simulink model "mrefrobotarm_modified_previous_y_previous_u_previous_ref_pert_2"  (R2018b)
settings: Solver=FixedStepAuto  StartTime=0.0  StopTime=60  RelTol=1e-3  AbsTol=1e-6
undefined symbols (not defined in the file or in its folder): cc, options
libraries: neural x858, simulink x1
(part 24 of 32)

== system mrefrobotarm_modified_previous_y_previous_u_previous_ref_pert_2/m=0.001 sd=0.001/Layer 3/Delays 1 ==
  "p{3}" : Inport  PortDimensions=30
      mask Display: e = 0.06;c1 = [120 230 180]/255;c2 = ([120 230 180]+0)/(256+128);c3 = ([120 230 180]+128)/(256+128);patch([0 1 1 0],[0 0 1 1],c1);patch([0 1 1 1-e 1-e 0+e],[0 0 1 1-e 0+e 0+e],c2);patch([0 0 1 1-e 0+e 0+e],[0 1 1 1-e 1-e 0+e],c3);plot([0 1 1 0 0],[0 0 1 1 0]);
  mux : Mux  Inputs=1
      mask Display: e = 0.06;c1 = [120 150 230]/255;c2 = ([120 150 230]+0)/383;c3 = ([120 150 230]+128)/383;patch([0 1 1 0],[0 0 1 1],c1);patch([0 1 1 1-e 1-e 0+e],[0 0 1 1-e 0+e 0+e],c2);patch([0 0 1 1-e 0+e 0+e],[0 1 1 1-e 1-e 0+e],c3);plot([0 1 1 0 0],[0 0 1 1 0]);disp('Mux')
  "pd{3,2}" : Outport
      mask Display: e = 0.06;c1 = [120 230 180]/255;c2 = ([120 230 180]+0)/(256+128);c3 = ([120 230 180]+128)/(256+128);patch([0 1 1 0],[0 0 1 1],c1);patch([0 1 1 1-e 1-e 0+e],[0 0 1 1-e 0+e 0+e],c2);patch([0 0 1 1-e 0+e 0+e],[0 1 1 1-e 1-e 0+e],c3);plot([0 1 1 0 0],[0 0 1 1 0]);
  wires:
  "p{3}"/1 -> mux/1
  mux/1 -> "pd{3,2}"/1

== system mrefrobotarm_modified_previous_y_previous_u_previous_ref_pert_2/m=0.001 sd=0.001/Layer 3/LW{3,2} ==
  "ad{3,2}" : Inport  PortDimensions=30
      mask Display: e = 0.06;c1 = [120 230 180]/255;c2 = ([120 230 180]+0)/(256+128);c3 = ([120 230 180]+128)/(256+128);patch([0 1 1 0],[0 0 1 1],c1);patch([0 1 1 1-e 1-e 0+e],[0 0 1 1-e 0+e 0+e],c2);patch([0 0 1 1-e 0+e 0+e],[0 1 1 1-e 1-e 0+e],c3);plot([0 1 1 0 0],[0 0 1 1 0]);
  "IW{3,2}(1,:)'" : Constant  Value=[-0.00096598592137593663510541919237084584892727434635162353515625;-0.03126267992859599331723075010813772678375244140625;-0.00195354501463004294470326982491314993239939212799072265625;-0.047903518138686769500811379884908092208206653594970703125;-0.0230636981987975865637796601959053077735006809234619140625;0.1680979203439105507111861470548319630324840545654296875;-0.0023952928575741243809316127766351200989447534084320068359375;0.0088298450217599577793947673853836022317409515380859375;0.00448404494478483149622061176842180429957807064056396484375;0.07350633081296938098336823941281181760132312774658203125;0.004624123527908109536344039014466034132055938243865966796875;0.03743489095666606425449884909539832733571529388427734375;-0.12573771491850338488660554503439925611019134521484375;-0.07859633251545668219950613320179400034248828887939453125;0.005914082534642393917945213388520642183721065521240234375;0.0135763042468372945037469179396794061176478862762451171875;0.0154239171401948822748284584349676151759922504425048828125;-0.007373815499766849142215807688671702635474503040313720703125;0.001608015075631823685708976512387380353175103664398193359375;0.0603517965756205920779819962262990884482860565185546875;-0.77977075469641288218980434976401738822460174560546875;0.85569988582330436255318772964528761804103851318359375;0.01259027748586210616876801537955543608404695987701416015625;-0.003409584380003004115688991504384830477647483348846435546875;-0.03508176609962354586258470590109936892986297607421875;0.0153176587784085542487400033451194758526980876922607421875;0.053023670382310893189892198051893501542508602142333984375;-0.0218811595943164440003503301568343886174261569976806640625;-0.0679133358367276229738962456394801847636699676513671875;0.1352169568786299180818133436332573182880878448486328125]
      mask Display: e = 0.06;c1 = [120 150 230]/255;c2 = ([120 150 230]+0)/383;c3 = ([120 150 230]+128)/383;patch([0 1 1 0],[0 0 1 1],c1);patch([0 1 1 1-e 1-e 0+e],[0 0 1 1-e 0+e 0+e],c2);patch([0 0 1 1-e 0+e 0+e],[0 1 1 1-e 1-e 0+e],c3);plot([0 1 1 0 0],[0 0 1 1 0]);disp('weights');
  Mux : Mux  Inputs=1
      mask Display: e = 0.06;c1 = [120 150 230]/255;c2 = ([120 150 230]+0)/383;c3 = ([120 150 230]+128)/383;patch([0 1 1 0],[0 0 1 1],c1);patch([0 1 1 1-e 1-e 0+e],[0 0 1 1-e 0+e 0+e],c2);patch([0 0 1 1-e 0+e 0+e],[0 1 1 1-e 1-e 0+e],c3);plot([0 1 1 0 0],[0 0 1 1 0]);disp('Mux');
  dotprod1 : neural/Weight Functions/dotprod
  "lz{3,2}" : Outport
      mask Display: e = 0.06;c1 = [120 230 180]/255;c2 = ([120 230 180]+0)/(256+128);c3 = ([120 230 180]+128)/(256+128);patch([0 1 1 0],[0 0 1 1],c1);patch([0 1 1 1-e 1-e 0+e],[0 0 1 1-e 0+e 0+e],c2);patch([0 0 1 1-e 0+e 0+e],[0 1 1 1-e 1-e 0+e],c3);plot([0 1 1 0 0],[0 0 1 1 0]);
  wires:
  "IW{3,2}(1,:)'"/1 -> dotprod1/1
  "ad{3,2}"/1 -> dotprod1/2
  dotprod1/1 -> Mux/1
  Mux/1 -> "lz{3,2}"/1

== system mrefrobotarm_modified_previous_y_previous_u_previous_ref_pert_2/m=0.001 sd=0.001 unclear/Layer 1/Delays 1 ==
  "p{1}" : Inport  PortDimensions=10
      mask Display: e = 0.06;c1 = [120 230 180]/255;c2 = ([120 230 180]+0)/(256+128);c3 = ([120 230 180]+128)/(256+128);patch([0 1 1 0],[0 0 1 1],c1);patch([0 1 1 1-e 1-e 0+e],[0 0 1 1-e 0+e 0+e],c2);patch([0 0 1 1-e 0+e 0+e],[0 1 1 1-e 1-e 0+e],c3);plot([0 1 1 0 0],[0 0 1 1 0]);
  mux : Mux  Inputs=1
      mask Display: e = 0.06;c1 = [120 150 230]/255;c2 = ([120 150 230]+0)/383;c3 = ([120 150 230]+128)/383;patch([0 1 1 0],[0 0 1 1],c1);patch([0 1 1 1-e 1-e 0+e],[0 0 1 1-e 0+e 0+e],c2);patch([0 0 1 1-e 0+e 0+e],[0 1 1 1-e 1-e 0+e],c3);plot([0 1 1 0 0],[0 0 1 1 0]);disp('Mux')
  "pd{1,1}" : Outport
      mask Display: e = 0.06;c1 = [120 230 180]/255;c2 = ([120 230 180]+0)/(256+128);c3 = ([120 230 180]+128)/(256+128);patch([0 1 1 0],[0 0 1 1],c1);patch([0 1 1 1-e 1-e 0+e],[0 0 1 1-e 0+e 0+e],c2);patch([0 0 1 1-e 0+e 0+e],[0 1 1 1-e 1-e 0+e],c3);plot([0 1 1 0 0],[0 0 1 1 0]);
  wires:
  "p{1}"/1 -> mux/1
  mux/1 -> "pd{1,1}"/1

== system mrefrobotarm_modified_previous_y_previous_u_previous_ref_pert_2/m=0.001 sd=0.001 unclear/Layer 1/IW{1,1} ==
  "pd{1,1}" : Inport  PortDimensions=10
      mask Display: e = 0.06;c1 = [120 230 180]/255;c2 = ([120 230 180]+0)/(256+128);c3 = ([120 230 180]+128)/(256+128);patch([0 1 1 0],[0 0 1 1],c1);patch([0 1 1 1-e 1-e 0+e],[0 0 1 1-e 0+e 0+e],c2);patch([0 0 1 1-e 0+e 0+e],[0 1 1 1-e 1-e 0+e],c3);plot([0 1 1 0 0],[0 0 1 1 0]);
  "IW{1,1}(1,:)'" : Constant  Value=[0.350735520146514712092056242909166030585765838623046875;-0.365382843268743207065796241295174695551395416259765625;-0.99622776359163045523104074163711629807949066162109375;-0.2204237782535651835047474378370679914951324462890625;-1.1029132366021070499328970981878228485584259033203125;0.1267678513277864238428804810610017739236354827880859375;0.11285976385185104986508264346412033773958683013916015625;0.0266590202247262118839810085546560003422200679779052734375;1.4467040095656533704726598443812690675258636474609375;1.3454075388999766627051712930551730096340179443359375]
      mask Display: e = 0.06;c1 = [120 150 230]/255;c2 = ([120 150 230]+0)/383;c3 = ([120 150 230]+128)/383;patch([0 1 1 0],[0 0 1 1],c1);patch([0 1 1 1-e 1-e 0+e],[0 0 1 1-e 0+e 0+e],c2);patch([0 0 1 1-e 0+e 0+e],[0 1 1 1-e 1-e 0+e],c3);plot([0 1 1 0 0],[0 0 1 1 0]);disp('Weights');
  "IW{1,1}(10,:)'" : Constant  Value=[0.489180396685796214928387826148536987602710723876953125;0.025688296059734945508967740579464589245617389678955078125;-0.8253001755471967015864720451645553112030029296875;-0.3423875044746698126374440107611007988452911376953125;2.30371194741592777432970251538790762424468994140625;-3.4241648689344543754486949183046817779541015625;1.3873334301899580278671919586486183106899261474609375;-0.44829248082369443917372109353891573846340179443359375;-0.584485848536391738861084377276711165904998779296875;-0.78044816092502511395423425710760056972503662109375]
      mask Display: e = 0.06;c1 = [120 150 230]/255;c2 = ([120 150 230]+0)/383;c3 = ([120 150 230]+128)/383;patch([0 1 1 0],[0 0 1 1],c1);patch([0 1 1 1-e 1-e 0+e],[0 0 1 1-e 0+e 0+e],c2);patch([0 0 1 1-e 0+e 0+e],[0 1 1 1-e 1-e 0+e],c3);plot([0 1 1 0 0],[0 0 1 1 0]);disp('Weights');
  "IW{1,1}(11,:)'" : Constant  Value=[0.18698885547596300060746443705284036695957183837890625;0.93870062216768701546243391931056976318359375;-0.87771687606838610928861044158111326396465301513671875;0.525629157232238686248138037626631557941436767578125;-0.584803275112354636888767345226369798183441162109375;-0.78398570882191587205767291379743255674839019775390625;-0.6750269388772991430158754155854694545269012451171875;-0.037333925850436155968736784416250884532928466796875;-1.1760354680013247463676862025749869644641876220703125;-0.3408361228029785916504579290631227195262908935546875]
      mask Display: e = 0.06;c1 = [120 150 230]/255;c2 = ([120 150 230]+0)/383;c3 = ([120 150 230]+128)/383;patch([0 1 1 0],[0 0 1 1],c1);patch([0 1 1 1-e 1-e 0+e],[0 0 1 1-e 0+e 0+e],c2);patch([0 0 1 1-e 0+e 0+e],[0 1 1 1-e 1-e 0+e],c3);plot([0 1 1 0 0],[0 0 1 1 0]);disp('Weights');
  "IW{1,1}(12,:)'" : Constant  Value=[0.0215852682713452322105229796989078749902546405792236328125;-0.51872830046918327884242216896382160484790802001953125;-0.468248523931060589564623342084814794361591339111328125;-0.50647243936863173274787186528556048870086669921875;-0.78157350595780050728222931866184808313846588134765625;3.41692574461050213585622259415686130523681640625;-2.23846059049971923826660713530145585536956787109375;-0.60927422485717841471597466806997545063495635986328125;0.29327799124264597452338421135209500789642333984375;0.08903506975016380053933318095005233772099018096923828125]
      mask Display: e = 0.06;c1 = [120 150 230]/255;c2 = ([120 150 230]+0)/383;c3 = ([120 150 230]+128)/383;patch([0 1 1 0],[0 0 1 1],c1);patch([0 1 1 1-e 1-e 0+e],[0 0 1 1-e 0+e 0+e],c2);patch([0 0 1 1-e 0+e 0+e],[0 1 1 1-e 1-e 0+e],c3);plot([0 1 1 0 0],[0 0 1 1 0]);disp('Weights');
  "IW{1,1}(13,:)'" : Constant  Value=[0.6746875013157798139928900127415545284748077392578125;-0.62489238655318668502758328031632117927074432373046875;0.1629262490629680704135040514302090741693973541259765625;-0.1367019703160116950169111760260420851409435272216796875;-0.75570950017347160443392795059480704367160797119140625;2.003318792327748010251298182993195950984954833984375;-1.1536359129580089355471272938302718102931976318359375;-0.041927729311054200145303383351347292773425579071044921875;0.843791037259761456112983069033361971378326416015625;1.0843679220652264749702453627833165228366851806640625]
      mask Display: e = 0.06;c1 = [120 150 230]/255;c2 = ([120 150 230]+0)/383;c3 = ([120 150 230]+128)/383;patch([0 1 1 0],[0 0 1 1],c1);patch([0 1 1 1-e 1-e 0+e],[0 0 1 1-e 0+e 0+e],c2);patch([0 0 1 1-e 0+e 0+e],[0 1 1 1-e 1-e 0+e],c3);plot([0 1 1 0 0],[0 0 1 1 0]);disp('Weights');
  "IW{1,1}(14,:)'" : Constant  Value=[0.1064105997657826818691972903252462856471538543701171875;-0.76827006137680131647726966548361815512180328369140625;1.186307378378237853411292235250584781169891357421875;0.56761102937644825061624942463822662830352783203125;-1.5212597719010518826365796485333703458309173583984375;1.5024445400946202511249794042669236660003662109375;-1.3109166464008394914486643756390549242496490478515625;0.08636767886193663645855167487752623856067657470703125;-1.7985044176385340808366208875668235123157501220703125;-0.31523953859487263695626779735903255641460418701171875]
      mask Display: e = 0.06;c1 = [120 150 230]/255;c2 = ([120 150 230]+0)/383;c3 = ([120 150 230]+128)/383;patch([0 1 1 0],[0 0 1 1],c1);patch([0 1 1 1-e 1-e 0+e],[0 0 1 1-e 0+e 0+e],c2);patch([0 0 1 1-e 0+e 0+e],[0 1 1 1-e 1-e 0+e],c3);plot([0 1 1 0 0],[0 0 1 1 0]);disp('Weights');
  "IW{1,1}(15,:)'" : Constant  Value=[-0.281470768776616087070152616433915682137012481689453125;1.3938473337264507545540936916950158774852752685546875;-1.0094685935062079895629949533031322062015533447265625;-0.462216053281385708118023103452287614345550537109375;-2.023964996515461134407587451278232038021087646484375;0.488549499659554575803355191965238191187381744384765625;0.67736367905604721872947493466199375689029693603515625;0.340098821019820307665071368319331668317317962646484375;0.82710042766707292383188132589566521346569061279296875;0.03264495933566601004738316760267480276525020599365234375]
      mask Display: e = 0.06;c1 = [120 150 230]/255;c2 = ([120 150 230]+0)/383;c3 = ([120 150 230]+128)/383;patch([0 1 1 0],[0 0 1 1],c1);patch([0 1 1 1-e 1-e 0+e],[0 0 1 1-e 0+e 0+e],c2);patch([0 0 1 1-e 0+e 0+e],[0 1 1 1-e 1-e 0+e],c3);plot([0 1 1 0 0],[0 0 1 1 0]);disp('Weights');
  "IW{1,1}(16,:)'" : Constant  Value=[0.51236814799393159969298494615941308438777923583984375;-0.11271288636420510875790768068327452056109905242919921875;-0.86745597821140341121548544833785854279994964599609375;-0.0444761804672831051465919927068171091377735137939453125;0.292548210338565983779091084215906448662281036376953125;1.1887786529416064507103101277607493102550506591796875;-1.5965228644647548872370634853723458945751190185546875;-0.1933031790978570196859465113448095507919788360595703125;1.653612394779674144018599690753035247325897216796875;1.692624596770178957427788191125728189945220947265625]
      mask Display: e = 0.06;c1 = [120 150 230]/255;c2 = ([120 150 230]+0)/383;c3 = ([120 150 230]+128)/383;patch([0 1 1 0],[0 0 1 1],c1);patch([0 1 1 1-e 1-e 0+e],[0 0 1 1-e 0+e 0+e],c2);patch([0 0 1 1-e 0+e 0+e],[0 1 1 1-e 1-e 0+e],c3);plot([0 1 1 0 0],[0 0 1 1 0]);disp('Weights');
  "IW{1,1}(17,:)'" : Constant  Value=[-0.134713277390601182670337720992392860352993011474609375;-0.219753726466271059880597249502898193895816802978515625;-0.97312594474185909465546728824847377836704254150390625;-0.97666131491126095820476393782882951200008392333984375;1.6758765760164207048177331671467982232570648193359375;1.6573586744697614836496768475626595318317413330078125;-2.5128893468034192437698948197066783905029296875;-1.038259378285322664936529690749011933803558349609375;-0.2440796527404064109045833674827008508145809173583984375;-0.2393407823319994298660873255357728339731693267822265625]
      mask Display: e = 0.06;c1 = [120 150 230]/255;c2 = ([120 150 230]+0)/383;c3 = ([120 150 230]+128)/383;patch([0 1 1 0],[0 0 1 1],c1);patch([0 1 1 1-e 1-e 0+e],[0 0 1 1-e 0+e 0+e],c2);patch([0 0 1 1-e 0+e 0+e],[0 1 1 1-e 1-e 0+e],c3);plot([0 1 1 0 0],[0 0 1 1 0]);disp('Weights');
  "IW{1,1}(18,:)'" : Constant  Value=[0.99551000395831923395206786153721623122692108154296875;0.309330504610104084495247889208258129656314849853515625;0.0982691280072249540022966129981796257197856903076171875;0.09682416435452499692271288722622557543218135833740234375;-0.230335024806646859740766331015038304030895233154296875;-1.54776210110588241519735674955882132053375244140625;1.1727252690063643125739645256544463336467742919921875;-0.173263109696820405414285914957872591912746429443359375;-0.320343827491524402173439511898322962224483489990234375;0.2498583383515806388697200191018055193126201629638671875]
      mask Display: e = 0.06;c1 = [120 150 230]/255;c2 = ([120 150 230]+0)/383;c3 = ([120 150 230]+128)/383;patch([0 1 1 0],[0 0 1 1],c1);patch([0 1 1 1-e 1-e 0+e],[0 0 1 1-e 0+e 0+e],c2);patch([0 0 1 1-e 0+e 0+e],[0 1 1 1-e 1-e 0+e],c3);plot([0 1 1 0 0],[0 0 1 1 0]);disp('Weights');
  "IW{1,1}(19,:)'" : Constant  Value=[0.76429313189230752012548464335850439965724945068359375;-0.521540128957617366012300408328883349895477294921875;0.3915818297651803003844861450488679111003875732421875;0.63022242812250706123222698806785047054290771484375;-0.2425709596863108996611657630637637339532375335693359375;0.91759977645770918197598575716256164014339447021484375;-1.8532788341151775757253972187754698097705841064453125;0.599831021911985562411473438260145485401153564453125;-0.81235773591966620177373670230736024677753448486328125;0.322657045127163921716118011318030767142772674560546875]
      mask Display: e = 0.06;c1 = [120 150 230]/255;c2 = ([120 150 230]+0)/383;c3 = ([120 150 230]+128)/383;patch([0 1 1 0],[0 0 1 1],c1);patch([0 1 1 1-e 1-e 0+e],[0 0 1 1-e 0+e 0+e],c2);patch([0 0 1 1-e 0+e 0+e],[0 1 1 1-e 1-e 0+e],c3);plot([0 1 1 0 0],[0 0 1 1 0]);disp('Weights');
  "IW{1,1}(2,:)'" : Constant  Value=[0.82340518925201855449103049977566115558147430419921875;0.68418765412697502004135685638175345957279205322265625;-0.8501983817765752515782651244080625474452972412109375;-0.6725354241137353472623772177030332386493682861328125;-1.686489839770609844293858259334228932857513427734375;0.02659254733545494964186417519158567301928997039794921875;1.369605202314759129222920819302089512348175048828125;0.366403171174389974407148429236258380115032196044921875;-1.3169485462379999507476213693735189735889434814453125;-0.7536444755594915445584547342150472104549407958984375]
      mask Display: e = 0.06;c1 = [120 150 230]/255;c2 = ([120 150 230]+0)/383;c3 = ([120 150 230]+128)/383;patch([0 1 1 0],[0 0 1 1],c1);patch([0 1 1 1-e 1-e 0+e],[0 0 1 1-e 0+e 0+e],c2);patch([0 0 1 1-e 0+e 0+e],[0 1 1 1-e 1-e 0+e],c3);plot([0 1 1 0 0],[0 0 1 1 0]);disp('Weights');
  "IW{1,1}(20,:)'" : Constant  Value=[-0.447015034910001995971384758377098478376865386962890625;0.149185741272195471207595574014703743159770965576171875;-0.87865230831664853372586776458774693310260772705078125;-0.59172904119554825541626996709965169429779052734375;-0.9017728117737029425171613183920271694660186767578125;-0.5286866174093571846270833702874369919300079345703125;0.1539000184345160338050817472321796230971813201904296875;-0.09933451350243531485784131973559851758182048797607421875;0.345969916904256435952191850446979515254497528076171875;-0.68540991998586975331164694580365903675556182861328125]
      mask Display: e = 0.06;c1 = [120 150 230]/255;c2 = ([120 150 230]+0)/383;c3 = ([120 150 230]+128)/383;patch([0 1 1 0],[0 0 1 1],c1);patch([0 1 1 1-e 1-e 0+e],[0 0 1 1-e 0+e 0+e],c2);patch([0 0 1 1-e 0+e 0+e],[0 1 1 1-e 1-e 0+e],c3);plot([0 1 1 0 0],[0 0 1 1 0]);disp('Weights');
  "IW{1,1}(21,:)'" : Constant  Value=[-0.97062112534156586018951884398120455443859100341796875;-0.782595078403797383970186274382285773754119873046875;0.8959050885798418573102708251099102199077606201171875;-0.7204804251835532635794834277476184070110321044921875;1.3827696031012930433234942029230296611785888671875;0.87714097058526940831058027470135129988193511962890625;-0.058464479317534810698386849026064737699925899505615234375;-0.6598280166511683031416168887517414987087249755859375;1.0607038212290424983308412265614606440067291259765625;-0.011389639449299278350924424785262090153992176055908203125]
      mask Display: e = 0.06;c1 = [120 150 230]/255;c2 = ([120 150 230]+0)/383;c3 = ([120 150 230]+128)/383;patch([0 1 1 0],[0 0 1 1],c1);patch([0 1 1 1-e 1-e 0+e],[0 0 1 1-e 0+e 0+e],c2);patch([0 0 1 1-e 0+e 0+e],[0 1 1 1-e 1-e 0+e],c3);plot([0 1 1 0 0],[0 0 1 1 0]);disp('Weights');
  "IW{1,1}(22,:)'" : Constant  Value=[0.414146735253828335299175478212418965995311737060546875;0.481767503224955373486437792962533421814441680908203125;-0.62951020673122404236465854410198517143726348876953125;-0.39212331166395575365868353401310741901397705078125;0.419185550868260314860691551075433380901813507080078125;-0.0646730718021691630692515673217712901532649993896484375;-0.6080676876355710636090634579886682331562042236328125;0.86781010731096064336753670431789942085742950439453125;-0.1751497710579812683295841679864679463207721710205078125;-1.19956254116058769199071321054361760616302490234375]
      mask Display: e = 0.06;c1 = [120 150 230]/255;c2 = ([120 150 230]+0)/383;c3 = ([120 150 230]+128)/383;patch([0 1 1 0],[0 0 1 1],c1);patch([0 1 1 1-e 1-e 0+e],[0 0 1 1-e 0+e 0+e],c2);patch([0 0 1 1-e 0+e 0+e],[0 1 1 1-e 1-e 0+e],c3);plot([0 1 1 0 0],[0 0 1 1 0]);disp('Weights');
  "IW{1,1}(23,:)'" : Constant  Value=[0.63927426416386856633522484116838313639163970947265625;-0.886834589506090953392458686721511185169219970703125;0.064777683987573830837192190301720984280109405517578125;-0.12250510452413461426335317128177848644554615020751953125;-1.3690684671345765277550299288122914731502532958984375;1.548769536535032020907465266645886003971099853515625;-0.212622841692526931556272984380484558641910552978515625;0.2278827500173041809006235780543647706508636474609375;-0.24529640546804498679733796961954794824123382568359375;0.0167355255684867414156524745294518652372062206268310546875]
      mask Display: e = 0.06;c1 = [120 150 230]/255;c2 = ([120 150 230]+0)/383;c3 = ([120 150 230]+128)/383;patch([0 1 1 0],[0 0 1 1],c1);patch([0 1 1 1-e 1-e 0+e],[0 0 1 1-e 0+e 0+e],c2);patch([0 0 1 1-e 0+e 0+e],[0 1 1 1-e 1-e 0+e],c3);plot([0 1 1 0 0],[0 0 1 1 0]);disp('Weights');
  "IW{1,1}(24,:)'" : Constant  Value=[-0.59744987564703533333698715068749152123928070068359375;-0.61217891723130579695322239786037243902683258056640625;-0.1463472385292276245483122920632013119757175445556640625;0.73567465684176436280239386178436689078807830810546875;0.375136908055977158493732304123113863170146942138671875;-0.66463862609319812602137744761421345174312591552734375;-1.12757765814861077302566627622582018375396728515625;0.09130206158397513593882877103169448673725128173828125;0.40718224827915550090295937479822896420955657958984375;0.1678970776673136822143561630582553334534168243408203125]
      mask Display: e = 0.06;c1 = [120 150 230]/255;c2 = ([120 150 230]+0)/383;c3 = ([120 150 230]+128)/383;patch([0 1 1 0],[0 0 1 1],c1);patch([0 1 1 1-e 1-e 0+e],[0 0 1 1-e 0+e 0+e],c2);patch([0 0 1 1-e 0+e 0+e],[0 1 1 1-e 1-e 0+e],c3);plot([0 1 1 0 0],[0 0 1 1 0]);disp('Weights');
  "IW{1,1}(25,:)'" : Constant  Value=[0.1822203219932407025627441043980070389807224273681640625;-0.74962198282031200502473211599863134324550628662109375;0.360769770139617473869719788126531057059764862060546875;0.03058100472812101677799745402808184735476970672607421875;0.07675659268147778935276193124082055874168872833251953125;0.94353579568672618638203175578382797539234161376953125;-0.73863043180200183002170888357795774936676025390625;-0.463413010444659045905524408226483501493930816650390625;-0.0783851508922373818588624772019102238118648529052734375;0.365542993545432348678758671667310409247875213623046875]
      mask Display: e = 0.06;c1 = [120 150 230]/255;c2 = ([120 150 230]+0)/383;c3 = ([120 150 230]+128)/383;patch([0 1 1 0],[0 0 1 1],c1);patch([0 1 1 1-e 1-e 0+e],[0 0 1 1-e 0+e 0+e],c2);patch([0 0 1 1-e 0+e 0+e],[0 1 1 1-e 1-e 0+e],c3);plot([0 1 1 0 0],[0 0 1 1 0]);disp('Weights');
  "IW{1,1}(26,:)'" : Constant  Value=[-0.08293379864700345382999557841685600578784942626953125;1.2654039981977296402959609622485004365444183349609375;0.29978111719239464161290698029915802180767059326171875;-0.72578508628124593915487139383913017809391021728515625;0.6643172908561567613361376061220653355121612548828125;0.5364343807740141745199480283190496265888214111328125;0.5681872234917701991463445665431208908557891845703125;-0.11077181766224390713215797177326749078929424285888671875;0.6197517547327964226866470198729075491428375244140625;-0.3649861380467875893174323209677822887897491455078125]
      mask Display: e = 0.06;c1 = [120 150 230]/255;c2 = ([120 150 230]+0)/383;c3 = ([120 150 230]+128)/383;patch([0 1 1 0],[0 0 1 1],c1);patch([0 1 1 1-e 1-e 0+e],[0 0 1 1-e 0+e 0+e],c2);patch([0 0 1 1-e 0+e 0+e],[0 1 1 1-e 1-e 0+e],c3);plot([0 1 1 0 0],[0 0 1 1 0]);disp('Weights');
  "IW{1,1}(27,:)'" : Constant  Value=[-0.445270570339922178160207977271056734025478363037109375;-0.3844654603981150220448625987046398222446441650390625;0.2081292349260845664371544216919573955237865447998046875;1.0487749065296638750766078373999334871768951416015625;-0.87694778451229649096632101645809598267078399658203125;-1.4520804210467461725642124292789958417415618896484375;0.44149383777287309893466726862243376672267913818359375;0.39423262513696866182755229601752944290637969970703125;-0.349495312241939470876417317413142882287502288818359375;0.54151288875565761760100258470629341900348663330078125]
      mask Display: e = 0.06;c1 = [120 150 230]/255;c2 = ([120 150 230]+0)/383;c3 = ([120 150 230]+128)/383;patch([0 1 1 0],[0 0 1 1],c1);patch([0 1 1 1-e 1-e 0+e],[0 0 1 1-e 0+e 0+e],c2);patch([0 0 1 1-e 0+e 0+e],[0 1 1 1-e 1-e 0+e],c3);plot([0 1 1 0 0],[0 0 1 1 0]);disp('Weights');
  "IW{1,1}(28,:)'" : Constant  Value=[-1.077772266625895980496352422051131725311279296875;0.73910703572368563474270786173292435705661773681640625;0.12127458273676593181189531378549872897565364837646484375;-0.5273204216158837720485053068841807544231414794921875;1.211684171418887512317041910137049853801727294921875;-1.1046145587607971716437305076397024095058441162109375;1.324486794041534576393814859329722821712493896484375;0.33312246979210169417484621590119786560535430908203125;-0.54487761318813310307263009235612116754055023193359375;-0.1506579505397783458331417705267085693776607513427734375]
      mask Display: e = 0.06;c1 = [120 150 230]/255;c2 = ([120 150 230]+0)/383;c3 = ([120 150 230]+128)/383;patch([0 1 1 0],[0 0 1 1],c1);patch([0 1 1 1-e 1-e 0+e],[0 0 1 1-e 0+e 0+e],c2);patch([0 0 1 1-e 0+e 0+e],[0 1 1 1-e 1-e 0+e],c3);plot([0 1 1 0 0],[0 0 1 1 0]);disp('Weights');
  "IW{1,1}(29,:)'" : Constant  Value=[-0.5240395826185435534938505952595733106136322021484375;0.739914785263013019545041970559395849704742431640625;-0.52232676514438336479173585757962428033351898193359375;-0.15882605914241398892272627563215792179107666015625;-0.168934994137417915371912613409222103655338287353515625;0.363289121404528791980936830441351048648357391357421875;1.4412340462629000814587243439746089279651641845703125;0.2237669808462975085117108164922683499753475189208984375;-0.52173785866068644878623672411777079105377197265625;0.92772438904896825651036351700895465910434722900390625]
      mask Display: e = 0.06;c1 = [120 150 230]/255;c2 = ([120 150 230]+0)/383;c3 = ([120 150 230]+128)/383;patch([0 1 1 0],[0 0 1 1],c1);patch([0 1 1 1-e 1-e 0+e],[0 0 1 1-e 0+e 0+e],c2);patch([0 0 1 1-e 0+e 0+e],[0 1 1 1-e 1-e 0+e],c3);plot([0 1 1 0 0],[0 0 1 1 0]);disp('Weights');
  "IW{1,1}(3,:)'" : Constant  Value=[0.11185429522417635050945960983881377615034580230712890625;0.523601371833942952349616462015546858310699462890625;-0.56985507775098398486335327106644399464130401611328125;-0.83293672910457139391127157068694941699504852294921875;0.1551775371999844777004540219422779045999050140380859375;-1.5293209587362930346188250041450373828411102294921875;1.1741548293898806942792134577757678925991058349609375;0.57906705496471910787903425443801097571849822998046875;-1.2018677568528435273265131399966776371002197265625;-0.94741243319685175539035526526276953518390655517578125]
      mask Display: e = 0.06;c1 = [120 150 230]/255;c2 = ([120 150 230]+0)/383;c3 = ([120 150 230]+128)/383;patch([0 1 1 0],[0 0 1 1],c1);patch([0 1 1 1-e 1-e 0+e],[0 0 1 1-e 0+e 0+e],c2);patch([0 0 1 1-e 0+e 0+e],[0 1 1 1-e 1-e 0+e],c3);plot([0 1 1 0 0],[0 0 1 1 0]);disp('Weights');
  "IW{1,1}(30,:)'" : Constant  Value=[1.668746567559152627069352092803455889225006103515625;-0.42867589761463154029996758254128508269786834716796875;-0.2382437224649456009029080405525746755301952362060546875;-0.5157914663799625376583435354405082762241363525390625;-0.913211230767515313999638237874023616313934326171875;0.1281070728078177178854701878663036040961742401123046875;-0.474678471410212854397769888237235136330127716064453125;0.8748627439690765950075501677929423749446868896484375;-0.068717740888597000914472801014198921620845794677734375;-0.376561738894475028782693470930098555982112884521484375]
      mask Display: e = 0.06;c1 = [120 150 230]/255;c2 = ([120 150 230]+0)/383;c3 = ([120 150 230]+128)/383;patch([0 1 1 0],[0 0 1 1],c1);patch([0 1 1 1-e 1-e 0+e],[0 0 1 1-e 0+e 0+e],c2);patch([0 0 1 1-e 0+e 0+e],[0 1 1 1-e 1-e 0+e],c3);plot([0 1 1 0 0],[0 0 1 1 0]);disp('Weights');
  "IW{1,1}(4,:)'" : Constant  Value=[0.626386916811764393742123502306640148162841796875;0.66355957008979504774259794430690817534923553466796875;-1.1758329665695439469885741345933638513088226318359375;-0.57759877919009039448638986868900246918201446533203125;0.2148432452029656047898242832161486148834228515625;-1.1395998983569046725250473173218779265880584716796875;0.396613453162261875295513391392887569963932037353515625;-0.9029734649571150573166278263670392334461212158203125;-1.003194440134803411268649142584763467311859130859375;-0.31618705827929238783013943248079158365726470947265625]
      mask Display: e = 0.06;c1 = [120 150 230]/255;c2 = ([120 150 230]+0)/383;c3 = ([120 150 230]+128)/383;patch([0 1 1 0],[0 0 1 1],c1);patch([0 1 1 1-e 1-e 0+e],[0 0 1 1-e 0+e 0+e],c2);patch([0 0 1 1-e 0+e 0+e],[0 1 1 1-e 1-e 0+e],c3);plot([0 1 1 0 0],[0 0 1 1 0]);disp('Weights');
  "IW{1,1}(5,:)'" : Constant  Value=[0.15235745223625773991926735106972046196460723876953125;0.04063536218788284248848441393420216627418994903564453125;-0.55671116367761641630096391963888891041278839111328125;0.11745390806188361898509953107350156642496585845947265625;0.56082800311731018094718592692515812814235687255859375;0.2126804250767819481904297163055161945521831512451171875;0.251625976250845539983203025258262641727924346923828125;-0.6763374200773391020646840843255631625652313232421875;0.261848725784636970903562769308337010443210601806640625;-0.660057056246898365969855149160139262676239013671875]
      mask Display: e = 0.06;c1 = [120 150 230]/255;c2 = ([120 150 230]+0)/383;c3 = ([120 150 230]+128)/383;patch([0 1 1 0],[0 0 1 1],c1);patch([0 1 1 1-e 1-e 0+e],[0 0 1 1-e 0+e 0+e],c2);patch([0 0 1 1-e 0+e 0+e],[0 1 1 1-e 1-e 0+e],c3);plot([0 1 1 0 0],[0 0 1 1 0]);disp('Weights');
  "IW{1,1}(6,:)'" : Constant  Value=[0.91938520303732562677367923242854885756969451904296875;-1.3259210412997646244548377580940723419189453125;-0.9567668490464582564669626663089729845523834228515625;-0.207397235785878375491364522531512193381786346435546875;0.06045317245114691095952963451054529286921024322509765625;-0.06705287941626243697346154704064247198402881622314453125;-0.09062226535478516697974527005499112419784069061279296875;0.293735746891927995694260289383237250149250030517578125;-1.11897188814837544867941687698476016521453857421875;-1.0012261665391519738221859370241872966289520263671875]
      mask Display: e = 0.06;c1 = [120 150 230]/255;c2 = ([120 150 230]+0)/383;c3 = ([120 150 230]+128)/383;patch([0 1 1 0],[0 0 1 1],c1);patch([0 1 1 1-e 1-e 0+e],[0 0 1 1-e 0+e 0+e],c2);patch([0 0 1 1-e 0+e 0+e],[0 1 1 1-e 1-e 0+e],c3);plot([0 1 1 0 0],[0 0 1 1 0]);disp('Weights');
  "IW{1,1}(7,:)'" : Constant  Value=[-0.75915789191661076085182457973132841289043426513671875;0.585538437283576573832988287904299795627593994140625;0.8699273326671403960830275536864064633846282958984375;1.0279837876319606326802613693871535360813140869140625;-0.59259310069970083656443193831364624202251434326171875;-0.2668187070617851208709225829807110130786895751953125;1.2108906767067935117410115708480589091777801513671875;0.63729733980704850182519294321537017822265625;-0.966450501674631201609599884250201284885406494140625;-0.025666554374464023435820081431302241981029510498046875]
      mask Display: e = 0.06;c1 = [120 150 230]/255;c2 = ([120 150 230]+0)/383;c3 = ([120 150 230]+128)/383;patch([0 1 1 0],[0 0 1 1],c1);patch([0 1 1 1-e 1-e 0+e],[0 0 1 1-e 0+e 0+e],c2);patch([0 0 1 1-e 0+e 0+e],[0 1 1 1-e 1-e 0+e],c3);plot([0 1 1 0 0],[0 0 1 1 0]);disp('Weights');
  "IW{1,1}(8,:)'" : Constant  Value=[-0.048217670968037674994466357247802079655230045318603515625;1.03317751204637975348532563657499849796295166015625;0.64271989566958975803601106235873885452747344970703125;0.24524652089011300670762238951283507049083709716796875;-0.011766424458269642006058575134375132620334625244140625;0.08041738801510252276916190794509020633995532989501953125;-0.09790581589764268954922954435460269451141357421875;0.9806434098621801265238673295243643224239349365234375;0.70598605076621290255189933304791338741779327392578125;-0.06003437287162827207254167660721577703952789306640625]
      mask Display: e = 0.06;c1 = [120 150 230]/255;c2 = ([120 150 230]+0)/383;c3 = ([120 150 230]+128)/383;patch([0 1 1 0],[0 0 1 1],c1);patch([0 1 1 1-e 1-e 0+e],[0 0 1 1-e 0+e 0+e],c2);patch([0 0 1 1-e 0+e 0+e],[0 1 1 1-e 1-e 0+e],c3);plot([0 1 1 0 0],[0 0 1 1 0]);disp('Weights');
  "IW{1,1}(9,:)'" : Constant  Value=[0.83752677380316520316938522228156216442584991455078125;-0.6488249053881298689105960875167511403560638427734375;-0.58667300722700321813363188994117081165313720703125;-0.671409684017666652522393633262254297733306884765625;0.5924651919913885844692913451581262052059173583984375;-0.1201322350770514801876487354093114845454692840576171875;-0.001404002309457380408275195549094860325567424297332763671875;-0.6285921811756141064364555859356187283992767333984375;0.389533221104397975320665636900230310857295989990234375;-0.06926122184120349356550860875358921475708484649658203125]
      mask Display: e = 0.06;c1 = [120 150 230]/255;c2 = ([120 150 230]+0)/383;c3 = ([120 150 230]+128)/383;patch([0 1 1 0],[0 0 1 1],c1);patch([0 1 1 1-e 1-e 0+e],[0 0 1 1-e 0+e 0+e],c2);patch([0 0 1 1-e 0+e 0+e],[0 1 1 1-e 1-e 0+e],c3);plot([0 1 1 0 0],[0 0 1 1 0]);disp('Weights');
  Mux : Mux  Inputs=30
      mask Display: e = 0.06;c1 = [120 150 230]/255;c2 = ([120 150 230]+0)/383;c3 = ([120 150 230]+128)/383;patch([0 1 1 0],[0 0 1 1],c1);patch([0 1 1 1-e 1-e 0+e],[0 0 1 1-e 0+e 0+e],c2);patch([0 0 1 1-e 0+e 0+e],[0 1 1 1-e 1-e 0+e],c3);plot([0 1 1 0 0],[0 0 1 1 0]);disp('Mux');
  dotprod{1..30} (30 alike) : neural/Weight Functions/dotprod
  "iz{1,1}" : Outport
      mask Display: e = 0.06;c1 = [120 230 180]/255;c2 = ([120 230 180]+0)/(256+128);c3 = ([120 230 180]+128)/(256+128);patch([0 1 1 0],[0 0 1 1],c1);patch([0 1 1 1-e 1-e 0+e],[0 0 1 1-e 0+e 0+e],c2);patch([0 0 1 1-e 0+e 0+e],[0 1 1 1-e 1-e 0+e],c3);plot([0 1 1 0 0],[0 0 1 1 0]);
  wires:
  "IW{1,1}(1,:)'"/1 -> dotprod1/1
  "pd{1,1}"/1 -> dotprod1/2, dotprod2/2, dotprod3/2, dotprod4/2, dotprod5/2, dotprod6/2, dotprod7/2, dotprod8/2, dotprod9/2, dotprod10/2, dotprod11/2, dotprod12/2, dotprod13/2, dotprod14/2, dotprod15/2, dotprod16/2, dotprod17/2, dotprod18/2, dotprod19/2, dotprod20/2, dotprod21/2, dotprod22/2, dotprod23/2, dotprod24/2, dotprod25/2, dotprod26/2, dotprod27/2, dotprod28/2, dotprod29/2, dotprod30/2
  dotprod1/1 -> Mux/1
  "IW{1,1}(2,:)'"/1 -> dotprod2/1
  dotprod2/1 -> Mux/2
  "IW{1,1}(3,:)'"/1 -> dotprod3/1
  dotprod3/1 -> Mux/3
  "IW{1,1}(4,:)'"/1 -> dotprod4/1
  dotprod4/1 -> Mux/4
  "IW{1,1}(5,:)'"/1 -> dotprod5/1
  dotprod5/1 -> Mux/5
  "IW{1,1}(6,:)'"/1 -> dotprod6/1
  dotprod6/1 -> Mux/6
  "IW{1,1}(7,:)'"/1 -> dotprod7/1
  dotprod7/1 -> Mux/7
  "IW{1,1}(8,:)'"/1 -> dotprod8/1
  dotprod8/1 -> Mux/8
  "IW{1,1}(9,:)'"/1 -> dotprod9/1
  dotprod9/1 -> Mux/9
  "IW{1,1}(10,:)'"/1 -> dotprod10/1
  dotprod10/1 -> Mux/10
  "IW{1,1}(11,:)'"/1 -> dotprod11/1
  dotprod11/1 -> Mux/11
  "IW{1,1}(12,:)'"/1 -> dotprod12/1
  dotprod12/1 -> Mux/12
  "IW{1,1}(13,:)'"/1 -> dotprod13/1
  dotprod13/1 -> Mux/13
  "IW{1,1}(14,:)'"/1 -> dotprod14/1
  dotprod14/1 -> Mux/14
  "IW{1,1}(15,:)'"/1 -> dotprod15/1
  dotprod15/1 -> Mux/15
  "IW{1,1}(16,:)'"/1 -> dotprod16/1
  dotprod16/1 -> Mux/16
  "IW{1,1}(17,:)'"/1 -> dotprod17/1
  dotprod17/1 -> Mux/17
  "IW{1,1}(18,:)'"/1 -> dotprod18/1
  dotprod18/1 -> Mux/18
  "IW{1,1}(19,:)'"/1 -> dotprod19/1
  dotprod19/1 -> Mux/19
  "IW{1,1}(20,:)'"/1 -> dotprod20/1
  dotprod20/1 -> Mux/20
  "IW{1,1}(21,:)'"/1 -> dotprod21/1
  dotprod21/1 -> Mux/21
  "IW{1,1}(22,:)'"/1 -> dotprod22/1
  dotprod22/1 -> Mux/22
  "IW{1,1}(23,:)'"/1 -> dotprod23/1
  dotprod23/1 -> Mux/23
  "IW{1,1}(24,:)'"/1 -> dotprod24/1
  dotprod24/1 -> Mux/24
  "IW{1,1}(25,:)'"/1 -> dotprod25/1
  dotprod25/1 -> Mux/25
  "IW{1,1}(26,:)'"/1 -> dotprod26/1
  dotprod26/1 -> Mux/26
  "IW{1,1}(27,:)'"/1 -> dotprod27/1
  dotprod27/1 -> Mux/27
  "IW{1,1}(28,:)'"/1 -> dotprod28/1
  dotprod28/1 -> Mux/28
  "IW{1,1}(29,:)'"/1 -> dotprod29/1
  dotprod29/1 -> Mux/29
  "IW{1,1}(30,:)'"/1 -> dotprod30/1
  dotprod30/1 -> Mux/30
  Mux/1 -> "iz{1,1}"/1

== system mrefrobotarm_modified_previous_y_previous_u_previous_ref_pert_2/m=0.001 sd=0.001 unclear/Layer 2/Delays 1 ==
  "p{2}" : Inport  PortDimensions=30
      mask Display: e = 0.06;c1 = [120 230 180]/255;c2 = ([120 230 180]+0)/(256+128);c3 = ([120 230 180]+128)/(256+128);patch([0 1 1 0],[0 0 1 1],c1);patch([0 1 1 1-e 1-e 0+e],[0 0 1 1-e 0+e 0+e],c2);patch([0 0 1 1-e 0+e 0+e],[0 1 1 1-e 1-e 0+e],c3);plot([0 1 1 0 0],[0 0 1 1 0]);
  mux : Mux  Inputs=1
      mask Display: e = 0.06;c1 = [120 150 230]/255;c2 = ([120 150 230]+0)/383;c3 = ([120 150 230]+128)/383;patch([0 1 1 0],[0 0 1 1],c1);patch([0 1 1 1-e 1-e 0+e],[0 0 1 1-e 0+e 0+e],c2);patch([0 0 1 1-e 0+e 0+e],[0 1 1 1-e 1-e 0+e],c3);plot([0 1 1 0 0],[0 0 1 1 0]);disp('Mux')
  "pd{2,1}" : Outport
      mask Display: e = 0.06;c1 = [120 230 180]/255;c2 = ([120 230 180]+0)/(256+128);c3 = ([120 230 180]+128)/(256+128);patch([0 1 1 0],[0 0 1 1],c1);patch([0 1 1 1-e 1-e 0+e],[0 0 1 1-e 0+e 0+e],c2);patch([0 0 1 1-e 0+e 0+e],[0 1 1 1-e 1-e 0+e],c3);plot([0 1 1 0 0],[0 0 1 1 0]);
  wires:
  "p{2}"/1 -> mux/1
  mux/1 -> "pd{2,1}"/1
